simulink model "NewCAN_4"  (R2021a)
settings: Solver=VariableStepAuto  StartTime=0.0  StopTime=5  RelTol=1e-2
values from neighbouring files (symbols this model uses):
  C = 1e-12    [newmain.m]
  Kidd1 = 0    [newmain.m]
  Kidi1 = 20    [newmain.m]
  Kidi2 = 20    [newmain.m]
  Kidp1 = 5    [newmain.m]
  Kiqd1 = 0    [newmain.m]
  Kiqi1 = 20    [newmain.m]
  Kiqi2 = 20    [newmain.m]
  Kiqp1 = 5    [newmain.m]
  Kiqp2 = 5    [newmain.m]
  Kvdd = 0    [newmain.m]
  Kvdi = 40    [newmain.m]
  Kvdp = 10    [newmain.m]
  Kvqd = 0    [newmain.m]
  Kvqi = 40    [newmain.m]
  Kvqp = 10    [newmain.m]
  L = 100e-3    (= 0.1)    [newmain.m]
  Lf = 4e-3    (= 0.004)    [newmain.m]
  Ll = 31e-6    (= 3.1e-05)    [newmain.m]
  R = 4.33    [newmain.m]
  Rf = 40e-3    (= 0.04)    [newmain.m]
  RL = 0.1    [newmain.m]
  Rl = 0.1    [newmain.m]
  Ts = 0.51e-5    (= 5.1e-06)    [newmain.m]
undefined symbols (not defined in the file or in its folder): Ion, Lithium, sigbuilder_block
libraries: spsMeanLib x48, spsSeriesRLCBranchLib x13, pid_lib x12, spsFirstOrderFilterLib x8, spsIGBTDiodeLib x8, spsPWMGeneratorDCDCLib x8, spsabctodq0Lib x6, spsThreePhaseSeriesRLCBranchLib x4, spsThreePhaseVIMeasurementLib x4, truetime x3, spsdq0toAlphaBetaZeroLib x2, spsSVPWMGenerator2LevelLib x2
(part 3 of 3)

== system NewCAN_4/Microgrid Plant/Subsystem1/MPPT PnO ==
  V_PV : Inport
  I_PV : Inport  Port=2
  V_DC : Inport  Port=3
  SOC_B : Inport  Port=4
  Battery_scope 1 : Scope  NumInputPorts=4
  Compare To Constant : simulink/Logic and Bit Operations/Compare To Constant  Commented=on  relop=>=  const=98  OutDataTypeStr=boolean
  Constant : Constant  Value=1000
  From13 : From  Commented=on  GotoTag=D
  MATLAB Function : MATLAB Function  TreatAsAtomicUnit=on
  PID Controller : pid_lib/PID Controller  Controller=PI  Form=Parallel  TimeDomain=Continuous-time  UseExternalTs=off  SampleTime=-1  IntegratorMethod=Forward Euler  FilterMethod=Forward Euler  ControllerParametersSource=internal  P=1  I=1  D=0  UseFilter=on  N=100  TunerSelectOption=Transfer Function Based (PID Tuner App)  InitialConditionSource=internal  InitialConditionForIntegrator=0  InitialConditionForFilter=0  DifferentiatorICPrevScaledInput=0  ExternalReset=none  TrackingMode=off  Kt=1  LimitOutput=off  SatLimitsSource=internal  UpperSaturationLimit=inf  LowerSaturationLimit=-inf  LinearizeAsGain=on  AntiWindupMode=none  Kb=1  POutMin=[]  POutMax=[]  IOutMin=[]  IOutMax=[]  DOutMin=[]  DOutMax=[]  NOutMin=[]  NOutMax=[]  SumOutMin=[]  SumOutMax=[]  SaturationOutMin=[]  SaturationOutMax=[]  PParamMin=[]  PParamMax=[]  IParamMin=[]  IParamMax=[]  DParamMin=[]  DParamMax=[]  NParamMin=[]  NParamMax=[]  KbParamMin=[]  KbParamMax=[]  KtParamMin=[]  KtParamMax=[]  KbOutMin=[]  KbOutMax=[]  KtOutMin=[]  KtOutMax=[]  IntegratorOutMin=[]  IntegratorOutMax=[]  FilterOutMin=[]  FilterOutMax=[]  SumI1OutMin=[]  SumI1OutMax=[]  SumI2OutMin=[]  SumI2OutMax=[]  SumI3OutMin=[]  SumI3OutMax=[]  SumI4OutMin=[]  SumI4OutMax=[]  SumDOutMin=[]  SumDOutMax=[]  DifferentiatorOutMin=[]  DifferentiatorOutMax=[]  FilterDiffOutCoefMin=[]  FilterDiffOutCoefMax=[]  ReciprocalOutMin=[]  ReciprocalOutMax=[]  SumDenOutMin=[]  SumDenOutMax=[]  SumNumOutMin=[]  SumNumOutMax=[]  DivideOutMin=[]  DivideOutMax=[]  UdiffTsProdOutMin=[]  UdiffTsProdOutMax=[]  NTsProdOutMin=[]  NTsProdOutMax=[]  UintegralTsProdOutMin=[]  UintegralTsProdOutMax=[]  UngainTsProdOutMin=[]  UngainTsProdOutMax=[]  IntegratorContinuousStateAttributes=''  IntegratorStateMustResolveToSignalObject=off  IntegratorRTWStateStorageClass=Auto  FilterContinuousStateAttributes=''  FilterStateMustResolveToSignalObject=off  FilterRTWStateStorageClass=Auto  ParallelPVariant=InternalParameters  IdealPVariant=Disabled  IVariant=InternalParameters  DVariant=Disabled  IntegratorVariant=Continuous  SatVariant=Disabled  AWVariant=Passthrough  PCopyVariant=Disabled  TRVariant=Disabled  FdbkBlocksVariant=Forward  IdealPFdbkVariant=Disabled  SatFdbkVariant=Disabled  DerivativeFilterVariant=Disabled  NVariant=Disabled  NCopyVariant=Disabled_SignalSpec  FilterICVariant=Disabled  IntegratorICVariant=InternalICs  ExternalResetVariant=Disabled  TRSumVariant=Passthrough  SumFdbkVariant=Disabled  SumVariant=Sum_PI  TsampFilterVariant=InternalTs  TsampNgainVariant=Passthrough  TsampIntegralVariant=Passthrough  ExternalSaturationOutDataTypeStr=Inherit: Same as second input
  PWM Generator (DC-DC) : spsPWMGeneratorDCDCLib/PWM Generator (DC-DC)  Commented=on  Fsw=5000  Ts=0
  PWM Generator (DC-DC)1 : spsPWMGeneratorDCDCLib/PWM Generator (DC-DC)  Fsw=5000  Ts=0
  Saturation : Saturate
  Saturation1 : Saturate
  Sum : Sum  Inputs=|+-
  Switch : Switch  Criteria=u2 > Threshold
  D_PWM : Outport
  wires:
  PWM Generator (DC-DC)1/1 -> Switch/1
  PWM Generator (DC-DC)/1 -> Switch/3
  SOC_B/1 -> Compare To Constant/1
  Compare To Constant/1 -> Switch/2
  Saturation1/1 -> PWM Generator (DC-DC)1/1
  Switch/1 -> D_PWM/1
  PID Controller/1 -> Saturation1/1, Battery_scope 1/1
  Constant/1 -> Sum/1
  V_DC/1 -> Sum/2
  Sum/1 -> PID Controller/1, Battery_scope 1/2
  MATLAB Function/1(D) -> Saturation/1
  V_PV/1 -> MATLAB Function/1(Vpv)
  I_PV/1 -> MATLAB Function/2(Ipv)
  From13/1 -> PWM Generator (DC-DC)/1
  Saturation/1 -> [D]

== system NewCAN_4/Microgrid Plant/Subsystem1/Power Calculations ==
  V_Ba : Inport
  I_Ba : Inport  Port=2
  V_PV : Inport  Port=3
  I_PV : Inport  Port=4
  V_SC : Inport  Port=5
  I_SC : Inport  Port=6
  V_DC : Inport  Port=7
  I_Load : Inport  Port=8
  Mean{1..4} (4 alike) : spsMeanLib/Mean  Freq=60  Vinit=0  Ts=0
  Product{,1..3} (4 alike) : Product
  P_Ba : Outport
  P_PV : Outport  Port=2
  P_SC : Outport  Port=3
  P_Load : Outport  Port=4
  wires:
  Product1/1 -> Mean3/1
  Mean3/1 -> P_Load/1
  Product3/1 -> Mean2/1
  Mean2/1 -> P_SC/1
  Product/1 -> Mean1/1
  Mean1/1 -> P_PV/1
  Product2/1 -> Mean4/1
  Mean4/1 -> P_Ba/1
  I_SC/1 -> Product3/2
  V_SC/1 -> Product3/1
  I_Load/1 -> Product1/2
  V_DC/1 -> Product1/1
  I_PV/1 -> Product/2
  V_PV/1 -> Product/1
  V_Ba/1 -> Product2/1
  I_Ba/1 -> Product2/2

== system NewCAN_4/Microgrid Plant/Subsystem1/Signal Builder1 ==
  Demux : Demux  Tag=STV Demux  Outputs=2
      settings: DisplayOption=none
  FromWs : FromWorkspace  Tag=STV FromWs  VariableName=tuvar
      SigBuilderData=|
      | common.afterFinalStr = 'Extrapolate'
      | common.sampleTime = 0
      | dataSet.timeRange = [0 5]
      | dataSet.name = 'Group 1'
      | sbobj.Groups.Name = 'Group 1'
      | sbobj.Groups.Signals(1).Name = 'irradiance'
      | sbobj.Groups.Signals(1).XData = [0 1.505 1.505 5]
      | sbobj.Groups.Signals(1).YData = [1000 1000 950 798]
      | sbobj.Groups.Signals(2).Name = 'temp'
      | sbobj.Groups.Signals(2).XData = [0 2.75 5]
      | sbobj.Groups.Signals(2).YData = [25.98 25.48 24.5905882353]
      | sbobj.Groups.TimeRange = [0 5]
  irradiance : Outport  Tag=STV Outport
  temp : Outport  Tag=STV Outport  Port=2
  wires:
  FromWs/1 -> Demux/1
  Demux/1 -> irradiance/1
  Demux/2 -> temp/1

== matlab function NewCAN_4/Microgrid Plant/Subsystem1/MPPT PnO/MATLAB Function ==
  settings: updateMethod=DISCRETE  sampleTime=1e-4
  data: Vpv input; D output; Ipv input
function D = PandO(Vpv,Ipv)

persistent Dold Pold Vold


if isempty(Dold)
    Dold = 0.35;
    Vold = 17;
    Pold = 120;
end


deltaD = 0.001;

Ppv = Vpv*Ipv;

if (Ppv-Pold) ~= 0
    if (Ppv-Pold) > 0
        if (Vpv-Vold) > 0
            D = Dold - deltaD;
        else
            D = Dold + deltaD;
        end
    else
        if (Vpv-Vold) > 0
            D = Dold + deltaD;
        else
            D = Dold - deltaD;
        end        
    end
else
    D = Dold;
end

Dold = D;
Vold = Vpv;
Pold = Ppv;

== matlab function NewCAN_4/Microgrid Plant/Subsystem/MPPT PnO/MATLAB Function ==
  settings: updateMethod=DISCRETE  sampleTime=1e-4
  data: Vpv input; D output; Ipv input
function D = PandO(Vpv,Ipv)

persistent Dold Pold Vold


if isempty(Dold)
    Dold = 0.35;
    Vold = 29.5;
    Pold = 252.8;
end


deltaD = 0.001;

Ppv = Vpv*Ipv;

if (Ppv-Pold) ~= 0
    if (Ppv-Pold) > 0
        if (Vpv-Vold) > 0
            D = Dold - deltaD;
        else
            D = Dold + deltaD;
        end
    else
        if (Vpv-Vold) > 0
            D = Dold + deltaD;
        else
            D = Dold - deltaD;
        end        
    end
else
    D = Dold;
end

Dold = D;
Vold = Vpv;
Pold = Ppv;

== matlab function NewCAN_4/Microgrid Plant/Subsystem2/MATLAB Function ==
  data: ILd input; pL output; Vd input
function pL = fcn(ILd,Vd)

pL =3/2*(Vd*ILd);

== matlab function NewCAN_4/Microgrid Plant/Subsystem2/MATLAB Function1 ==
  data: ILq input; QL output; Vd input
function QL = fcn(ILq,Vd)

QL =-3/2*(Vd*ILq);

== matlab function NewCAN_4/Microgrid Plant/Subsystem3/MATLAB Function ==
  data: Itd_M input; p_M output; Vd input
function p_M = fcn(Itd_M,Vd)

p_M =3/2*(Vd*Itd_M);

== matlab function NewCAN_4/Microgrid Plant/Subsystem3/MATLAB Function1 ==
  data: Itq_M input; Q_M output; Vd input
function Q_M = fcn(Itq_M,Vd)

Q_M =-3/2*(Vd*Itq_M);

== matlab function NewCAN_4/Microgrid Plant/Subsystem4/MATLAB Function ==
  data: Itd_s input; p_S output; Vds input
function p_S = fcn(Itd_s,Vds)

p_S =3/2*(Vds*Itd_s);

== matlab function NewCAN_4/Microgrid Plant/POWER SHARING/power sharing1 ==
  data: Vir_star_d output; Itd_M input; Itd_s input
function Vir_star_d  = fcn(Itd_M,Itd_s)


 Vir_star_d = 1.33*(Itd_M + Itd_s )/2 ;

== matlab function NewCAN_4/Microgrid Plant/POWER SHARING/power sharing2 ==
  data: Vir_star_q output; Itq_M input; Itq_s input
function Vir_star_q  = fcn(Itq_M,Itq_s)


 Vir_star_q = 1.33*(Itq_M + Itq_s)/2 ;

== matlab function NewCAN_4/Microgrid Plant/Subsystem4/MATLAB Function1 ==
  data: Itq_s input; Q_S output; Vds input
function Q_S = fcn(Itq_s,Vds)

Q_S =-3/2*(Vds*Itq_s);
